simulink model "dc_motor_sim"  (R2021a)
settings: Solver=VariableStepAuto  StartTime=0.0  StopTime=10  MaxStep=1e-3  RelTol=1e-3
libraries: spsThyristorLib x4, spsSeriesRLCBranchLib x2, spsVoltageMeasurementLib x2, spspowerguiLib x1, spsACVoltageSourceLib x1
settings Model: Creator=AHMED  LastModifiedBy=AHMED

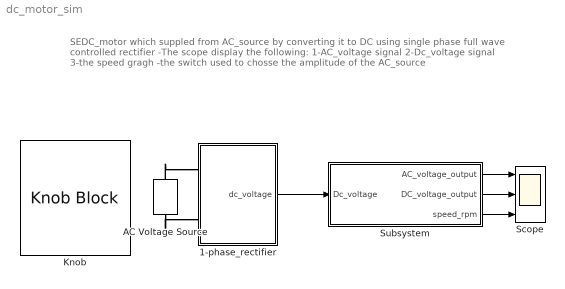
== system dc_motor_sim ==
  note: SEDC_motor which suppled from AC_source by converting it to DC using single phase full wave controlled rectifier
      | -The scope display the following:
      | 1-AC_voltage signal
      | 2-Dc_voltage signal
      | 3-the speed gragh
      | -the switch used to chosse the amplitude of the AC_source
  1-phase_rectifier : Subsystem
  AC Voltage Source : spsACVoltageSourceLib/AC Voltage Source  Amplitude=219.1071566180795  Phase=0  Frequency=2  SampleTime=0  Measurements=None  BusType=swing  Pref=10e3  Qref=0  Qmin=-inf  Qmax=+inf
  Knob : KnobBlock  ScaleMax=380
  Scope : Scope  NumInputPorts=3
  Subsystem : Subsystem  mask{Ra=0.5, La=0.1, Km=1.6, Kb=1.6, Tl=100, J=5, B=0.01}
  wires:
  Subsystem/3(speed_rpm) -> Scope/3
  1-phase_rectifier/1(dc_voltage) -> Subsystem/1(Dc_voltage)
  Subsystem/1(AC_voltage_output) -> Scope/1
  Subsystem/2(DC_voltage_output) -> Scope/2
  connections:
  AC Voltage Source/RConn1 -- 1-phase_rectifier/LConn1
  AC Voltage Source/LConn1 -- 1-phase_rectifier/LConn2

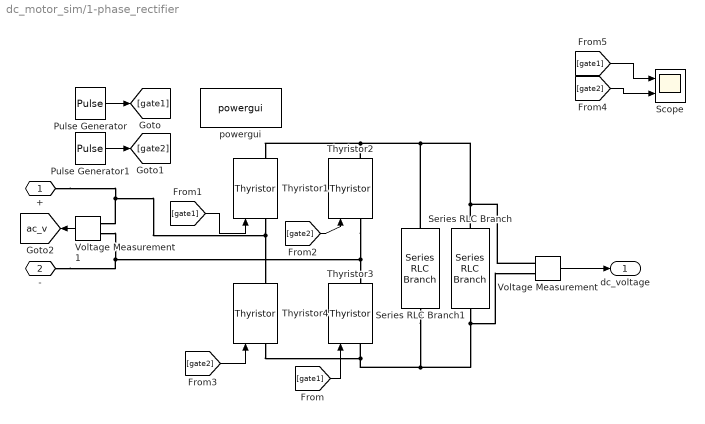
== system dc_motor_sim/1-phase_rectifier ==
  Pulse Generator : DiscretePulseGenerator  PulseType=Time based  Period=0.02  PulseWidth=5  PhaseDelay=0.0033
  Pulse Generator1 : DiscretePulseGenerator  PulseType=Time based  Period=0.02  PulseWidth=5  PhaseDelay=0.0133
  Scope : Scope  NumInputPorts=2
  Series RLC Branch : spsSeriesRLCBranchLib/Series RLC Branch  LConnTagsString=__new0  RConnTagsString=__new0  BranchType=R  Resistance=20  Inductance=1  SetiL0=off  InitialCurrent=0  Capacitance=1e-6  Setx0=off  InitialVoltage=0  Measurements=None
  Series RLC Branch1 : spsSeriesRLCBranchLib/Series RLC Branch  LConnTagsString=__new0  RConnTagsString=__new0  BranchType=C  Resistance=1  Inductance=1e-3  SetiL0=off  InitialCurrent=0  Capacitance=10e-3  Setx0=off  InitialVoltage=0  Measurements=None
  Thyristor{1..4} (4 alike) : spsThyristorLib/Thyristor  Ron=0.001  Lon=0  Vf=0.8  IC=0  Rs=500  Cs=250e-9  Measurements=on
  Voltage Measurement : spsVoltageMeasurementLib/Voltage Measurement  PhasorSimulation=off  OutputType=Complex  PSBequivalent=0
  Voltage Measurement1 : spsVoltageMeasurementLib/Voltage Measurement  PhasorSimulation=off  OutputType=Complex  PSBequivalent=0
  powergui : spspowerguiLib/powergui  Priority=1  SimulationMode=Continuous  SampleTime=50e-6  frequency=60  Iterations=50  frequencyindice=0  Pbase=100e6  ErrMax=1e-4  UnitsV=kV  UnitsW=MW  buscounter=0  FunctionMessages=off  echomessages=off  EnableUseOfTLC=off  CurrentSourceSwitches=off  DisableSnubberDevices=off  DisableRonSwitches=off  DisableVfSwitches=off  DisplayEquations=off  AutomaticDiscreteSolvers=off  SolverType=Tustin/Backward Euler (TBE)  Interpol=off  ExternalGateDelay=off  methode=off  Ts=100  x0status=blocks  SPID=on  SwTol=0  HookPort=off  NonlinearTolerance=1e-4  nMaxIteration=100  ContinueOnMaxIteration=off  RestoreLinks=warning  ResistiveCurrentMeasurement=off  Frange=[0:2:500]  Ylog=off  Xlog=on  ShowGrid=off  save=off  variable=ZData  structure=0  ZoomFFT=off  StartTime=0.0  cycles=1  DisplayStyle=1  fundamental=60  FreqAxis=off  MaxFrequency=1000  frequencyindicesteady=1  RmsSteady=1  display=off
  + : PMIOPort  Side=Left
  - : PMIOPort  Port=2  Side=Left
  dc_voltage : Outport
  tag scope: ac_v=global
  wires:
  Pulse Generator/1 -> [gate1]
  Pulse Generator1/1 -> [gate2]
  [gate1] -> Thyristor1/1
  [gate2] -> Thyristor4/1
  [gate1] -> Thyristor3/1
  [gate2] -> Thyristor2/1
  Voltage Measurement1/1 -> [ac_v]
  Voltage Measurement/1 -> dc_voltage/1
  [gate1] -> Scope/1
  [gate2] -> Scope/2
  connections:
  Thyristor4/LConn1 -- Voltage Measurement/LConn2 -- Series RLC Branch/RConn1 -- Series RLC Branch1/RConn1 -- Thyristor3/LConn1
  Series RLC Branch/LConn1 -- Voltage Measurement/LConn1 -- Series RLC Branch1/LConn1 -- Thyristor2/RConn1 -- Thyristor1/RConn1
  Thyristor2/LConn1 -- -/RConn1 -- Voltage Measurement1/LConn2 -- Thyristor3/RConn1
  Thyristor1/LConn1 -- +/RConn1 -- Voltage Measurement1/LConn1 -- Thyristor4/RConn1

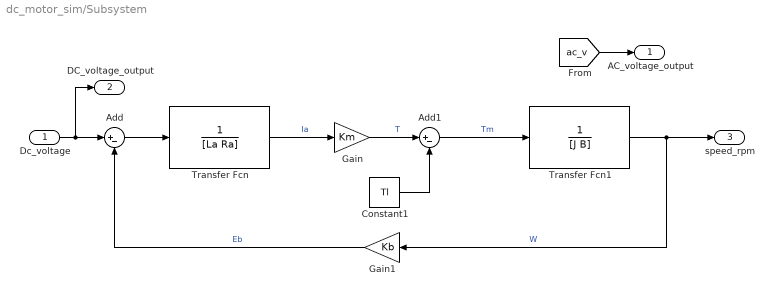
== system dc_motor_sim/Subsystem ==
  Dc_voltage : Inport
  Add : Sum  Inputs=|+-
  Add1 : Sum  Inputs=|+-
  Constant1 : Constant  Value=Tl
  Gain : Gain  Gain=Km
  Gain1 : Gain  Gain=Kb
  Transfer Fcn : TransferFcn  Denominator=[La Ra]
  Transfer Fcn1 : TransferFcn  Denominator=[J B]
  AC_voltage_output : Outport
  DC_voltage_output : Outport  Port=2
  speed_rpm : Outport  Port=3
  wires:
  Constant1/1 -> Add1/2
  Add1/1 -> Transfer Fcn1/1  "Tm"
  Transfer Fcn/1 -> Gain/1  "Ia"
  Gain1/1 -> Add/2  "Eb"
  Gain/1 -> Add1/1  "T"
  Add/1 -> Transfer Fcn/1
  Transfer Fcn1/1 -> speed_rpm/1, Gain1/1  "W"
  Dc_voltage/1 -> DC_voltage_output/1, Add/1
  [ac_v] -> AC_voltage_output/1
